simulink model "Commande_2_BackStepping"  (R2015a)
settings: Solver=ode3  StartTime=0.0  StopTime=5  FixedStep=0.0001  RelTol=1e-3
undefined symbols (not defined in the file or in its folder): sfun3d
(part 2 of 2)

== matlab function Commande_2_BackStepping/Point de Foncitonnement/T et ses derivees/Les matrices de lineairisation de d2P   ==
  data: P input; dP input; d2P input; d_d2P_alpha output; d_d2P_dalpha output; d_d2P_d2alpha output
    function [d_d2P_alpha, d_d2P_dalpha, d_d2P_d2alpha ]= fcn(P,dP,d2P)

    l1 = 0.19992; 
    l2 = 0.334; 
    r = 0.126; 
    phi2 = 2*pi/3;
    phi3 = 4*pi/3;

    %% Expression de P dans Ri
    % l'expression P1 dP1 et d2P1 ne se changent pas
    A2=[cos(phi2) sin(phi2) 0
        -sin(phi2) cos(phi2) 0
        0            0      1 ]; 
    A3=[cos(phi3) sin(phi3) 0
        -sin(phi3) cos(phi3) 0
        0            0      1 ];
     P2=A2*P; dP2=A2*dP; d2P2=A2*d2P; 
     P3=A3*P ; dP3=A3*dP ; d2P3=A3*d2P ; 
% Notation        
    x1=P(1); y1=P(2) ; z1=P(3) ; 
    x2=P2(1); y2=P2(2) ; z2=P2(3) ;
    x3=P3(1); y3=P3(2) ; z3=P3(3) ;

    %% Parametres du Triangle AiCiBi :
    % Triangle 1 :
    AB1=sqrt(z1^2+(x1-r)^2);
    e1=sqrt(l2^2-y1^2); 
    AB2=sqrt(z2^2+(x2-r)^2);
    e2=sqrt(l2^2-y2^2);
    AB3=sqrt(z3^2+(x3-r)^2);
    e3=sqrt(l2^2-y3^2);

% calcul de delta1
    delta1=acos((AB1^2 + l1^2 - e1^2)/(2*l1*AB1));
% calcul de delta2
    delta2=acos((AB2^2 + l1^2 - e2^2)/(2*l1*AB2));
% calcul de alpha3
    delta3=acos((AB3^2 + l1^2 - e3^2)/(2*l1*AB3));

%% =================== Calcule de dalpha_i ====================================

% ---------------------------- Calcul de dAlpha1 ----------------------
% Calcule de dDelta1 :
BH1 = AB1-l1*cos(delta1);
D1=l1*AB1*sin(delta1) ;
dDelta1X = -BH1*(x1-r)/AB1/D1 ; 
dDelta1Y = -y1/D1 ; 
dDelta1Z = -BH1*z1/AB1/D1 ; 
Gdelta1=  [ dDelta1X , dDelta1Y , dDelta1Z] ;
% Calcule de dBeta1 :
dBeta1Z=-(x1-r)/AB1^2 ; dBeta1X=z1/AB1^2 ;
Gbeta1=[ dBeta1X ,  0 , dBeta1Z] ;
% Calcule de dAlpha1 :
Galpha1=Gbeta1-Gdelta1 ;

% ---------------------------- Calcul de dAlpha2 ----------------------
% Calcule de dDelta2 :
BH2 = AB2-l1*cos(delta2);
D2=l1*AB2*sin(delta2) ;
dDelta2X = -BH2*(x2-r)/AB2/D2 ; 
dDelta2Y = -y2/D2 ; 
dDelta2Z = -BH2*z2/AB2/D2 ; 
Gdelta2=  [ dDelta2X , dDelta2Y , dDelta2Z] ;
% Calcule de dBeta2 :
dBeta2Z=-(x2-r)/AB2^2 ; dBeta2X=z2/AB2^2 ;
Gbeta2=[ dBeta2X ,  0 , dBeta2Z] ;
% Calcule de dAlpha2 :
Galpha2=Gbeta2-Gdelta2 ;

% ---------------------------- Calcul de dAlpha3 ----------------------
% Calcule de dDelta2 :
BH3 = AB3-l1*cos(delta3);
D3=l1*AB3*sin(delta3) ;
dDelta3X = -BH3*(x3-r)/AB3/D3 ; 
dDelta3Y = -y3/D3 ; 
dDelta3Z = -BH3*z3/AB3/D3 ; 
Gdelta3=  [ dDelta3X , dDelta3Y , dDelta3Z] ;
% Calcule de dBeta3:
dBeta3Z=-(x3-r)/AB3^2 ; dBeta2X=z3/AB3^2 ;
Gbeta3=[ dBeta2X ,  0 , dBeta3Z] ;
% Calcule de dAlpha3 :
Galpha3=Gbeta3-Gdelta3 ;

%% ===================== Calcule de d2alpha_i =================================
 
% ---------------------------- Calcul de d2Alpha1 ----------------------
% Calcule de d2Gama1 :
CH1=l1*sin(delta1);
AH1=l1*cos(delta1) ;
d2Delta1XX = -BH1*(x1-r)^2/(AB1^3*D1)*( AH1*e1^2/(BH1*CH1^2) + (AB1/(x1-r))^2 - 2 ) ;
d2Delta1YY = - (1+y1^2*AH1*AB1/D1^2 )  /D1;
d2Delta1ZZ  = -BH1*z1^2/(AB1^3*D1)*( AH1*e1^2/(BH1*CH1^2) + (AB1/z1)^2 -2 ) ;
d2Delta1XY = y1*(x1-r)*(CH1^2-AH1*BH1)/D1^3 ;
d2Delta1XZ = -BH1*(x1-r)*z1/(AB1^3*D1)*( AH1*e1^2/(BH1*CH1^2) - 2 ) ;
d2Delta1YZ = y1*z1*(CH1^2-AH1*BH1)/D1^3 ; 
Hdelta1=[ d2Delta1XX,d2Delta1XY,d2Delta1XZ ; d2Delta1XY, d2Delta1YY,d2Delta1YZ ;d2Delta1XZ , d2Delta1YZ,d2Delta1ZZ] ;
%Calcule de dBeta 1:
d2Beta1XX=-2*(x1-r)*z1/AB1^4 ; d2Beta1ZZ=-d2Beta1XX ; d2Beta1XZ = ((x1-r)^2-z1^2)/AB1^4 ;
Hbeta1= [d2Beta1XX , 0, d2Beta1XZ ; 0, 0, 0 ; d2Beta1XZ , 0 , d2Beta1ZZ ] ;
%Calcule de dAlpha1 :
Halpha1= Hbeta1 - Hdelta1; 

% ---------------------------- Calcul de d2Alpha2 ----------------------
% Calcule de d2Gama1 :
CH2=l1*sin(delta2);
AH2=l1*cos(delta2) ;
d2Delta2XX = -BH2*(x2-r)^2/(AB2^3*D2)*( AH2*e2^2/(BH2*CH2^2) + (AB2/(x2-r))^2 - 2 ) ;
d2Delta2YY = - (1+y2^2*AH2*AB2/D2^2 )  /D2;
d2Delta2ZZ  = -BH2*z2^2/(AB2^3*D2)*( AH2*e2^2/(BH2*CH2^2) + (AB2/z2)^2 -2 ) ;
d2Delta2XY = y2*(x2-r)*(CH2^2-AH2*BH2)/D2^3 ;
d2Delta2XZ = -BH2*(x2-r)*z2/(AB2^3*D2)*( AH2*e2^2/(BH2*CH2^2) - 2 ) ;
d2Delta2YZ = y2*z2*(CH2^2-AH2*BH2)/D2^3 ; 
Hdelta2=[ d2Delta2XX,d2Delta2XY,d2Delta2XZ ; d2Delta2XY, d2Delta2YY,d2Delta2YZ ;d2Delta2XZ , d2Delta2YZ,d2Delta2ZZ] ;
%Calcule de dBeta2:
d2Beta2XX=-2*(x2-r)*z2/AB2^4 ; d2Beta2ZZ=-d2Beta2XX ; d2Beta2XZ = ((x2-r)^2-z2^2)/AB2^4 ;
Hbeta2= [d2Beta2XX , 0, d2Beta2XZ ; 0, 0, 0 ; d2Beta2XZ , 0 , d2Beta2ZZ ] ;
%Calcule de dAlpha2 :
Halpha2= Hbeta2 - Hdelta2; 

% ---------------------------- Calcul de d2Alpha3 ----------------------
% Calcule de d2Gama3 :
CH3=l1*sin(delta3);
AH3=l1*cos(delta3) ;
d2Delta3XX = -BH3*(x3-r)^2/(AB3^3*D3)*( AH3*e3^2/(BH3*CH3^2) + (AB3/(x3-r))^2 - 2 ) ;
d2Delta3YY = - (1+y3^2*AH3*AB3/D3^2 )  /D3;
d2Delta3ZZ  = -BH3*z3^2/(AB3^3*D3)*( AH3*e3^2/(BH3*CH3^2) + (AB3/z3)^2 -2 ) ;
d2Delta3XY = y3*(x3-r)*(CH3^2-AH3*BH3)/D3^3 ;
d2Delta3XZ = -BH3*(x3-r)*z3/(AB3^3*D3)*( AH3*e3^2/(BH3*CH3^2) - 2 ) ;
d2Delta3YZ = y3*z3*(CH3^2-AH3*BH3)/D3^3 ; 
Hdelta3=[ d2Delta3XX,d2Delta3XY,d2Delta3XZ ; d2Delta3XY, d2Delta3YY,d2Delta3YZ ;d2Delta3XZ , d2Delta3YZ,d2Delta3ZZ] ;
%Calcule de dBeta3:
d2Beta3XX=-2*(x3-r)*z3/AB3^4 ; d2Beta3ZZ=-d2Beta3XX ; d2Beta3XZ = ((x3-r)^2-z3^2)/AB3^4 ;
Hbeta3= [d2Beta3XX , 0, d2Beta3XZ ; 0, 0, 0 ; d2Beta3XZ , 0 , d2Beta3ZZ ] ;
%Calcule de dAlpha3 :
Halpha3= Hbeta3 - Hdelta3; 

%% ==================== Caclcule de d3Alpahi ==================

%% ------------------------------ 1)  Calcule de d3Alpha1 -----------------------------
% Calcule de d3Delta1 :
% Parametres (1er derivees):
DH1=CH1^2-AH1*BH1 ;
dAB1X=(x1-r)/AB1 ; dAB1Z = z1/AB1 ; 
dD1X=(x1-r)*DH1/D1 ; dD1Z= z1*DH1/D1; dD1Y=-y1*AH1/CH1 ;
dAH1X=(x1-r)*BH1/AB1^2 ; dAH1Z = z1*BH1/AB1^2  ; 
dBH1X=(x1-r)*AH1/AB1^2 ; dBH1Z = z1*AH1/AB1^2  ; 
% Parametres (2eme derivees partielles):
% d2D1
d2D1XX=(DH1-(x1-r)^2-(dD1X)^2)/D1 ;
d2D1ZZ=(DH1-z1^2-(dD1Z)^2)/D1 ;
d2D1YY= -AH1/CH1-y1^2/D1*(1+(AH1/CH1)^2);
d2D1XZ = -(z1*(x1-r) + dD1X*dD1Z)/D1 ;
% d2AB1
d2AB1XX = 1/AB1 - (x1-r)*dAB1X/AB1^2 ;
d2AB1ZZ= 1/AB1 - z1*dAB1Z/AB1^2 ;
d2AB1XZ=-z1*(x1-r)/AB1^3;
%d2BH1
d2BH1ZZ=dBH1Z*(dAH1Z/AH1 +1/z1 - 2*dAB1Z/AB1) ;
d2BH1XX=dBH1X*(dAH1X/AH1 +1/(x1-r) - 2*dAB1X/AB1) ;
d2BH1XZ=z1*(x1-r)*(BH1-2*AH1)/AB1^4 ;

%------------------- les derivees partielles  d3Delta1_
d3Delta1ZZZ = d2Delta1ZZ*(dBH1Z/BH1+1/z1-dAB1Z/AB1-dD1Z/D1) + dDelta1Z*(-(dBH1Z/BH1)^2-1/z1^2+(dAB1Z/AB1)^2+(dD1Z/D1)^2 + d2BH1ZZ/BH1 - d2AB1ZZ/AB1 -d2D1ZZ/D1);
d3Delta1XXX = d2Delta1XX*(dBH1X/BH1+1/(x1-r)-dAB1X/AB1-dD1X/D1) + dDelta1X*(-(dBH1X/BH1)^2-1/(x1-r)^2+(dAB1X/AB1)^2+(dD1X/D1)^2 + d2BH1XX/BH1 - d2AB1XX/AB1 -d2D1XX/D1);
d3Delta1YYY= dD1Y/D1^2 + D1^2\(dD1Y + y1*d2D1YY-2*(dD1Y)^2*y1/D1);
d3Delta1XZZ= d2Delta1XZ*(dBH1Z/BH1+1/z1-dAB1Z/AB1-dD1Z/D1)+dDelta1Z*(-dBH1X*dBH1Z/BH1^2 + dAB1Z*dAB1X/AB1^2 + dD1Z*dD1X/D1^2 + d2BH1XZ/BH1 - d2AB1XZ/AB1 -d2D1XZ/D1) ;
d3Delta1XXZ= d2Delta1XZ*(dBH1X/BH1+1/(x1-r)-dAB1X/AB1-dD1X/D1)+dDelta1X*(-dBH1X*dBH1Z/BH1^2 + dAB1Z*dAB1X/AB1^2 + dD1Z*dD1X/D1^2 + d2BH1XZ/BH1 - d2AB1XZ/AB1 -d2D1XZ/D1) ;
d3Delta1XYY=(x1-r)/D1^3*(DH1-y1^2-3*y1*DH1*dD1Y/D1);
d3Delta1XXY=y1/D1^3*(DH1-(x1-r)^2*(1+3*(DH1/D1)^2));
d3Delta1YYZ=z1/D1^3*(DH1-y1^2-3*y1*DH1*dD1Y/D1);
d3Delta1YZZ=y1/D1^3*(DH1-z1^2*(1+3*(DH1/D1)^2));
d3Delta1XYZ=-(x1-r)*y1*z1/D1^3*(1+3*(DH1/D1)^2);
dHdelta1X=[ d3Delta1XXX,d3Delta1XXY,d3Delta1XXZ ; d3Delta1XXY, d3Delta1XYY,d3Delta1XYZ ;d3Delta1XXZ , d3Delta1XYZ,d3Delta1XZZ] ;
dHdelta1Y=[ d3Delta1XXY,d3Delta1XYY,d3Delta1XYZ ; d3Delta1XYY, d3Delta1YYY,d3Delta1YYZ ;d3Delta1XYZ , d3Delta1YYZ,d3Delta1YZZ] ;
dHdelta1Z=[ d3Delta1XXZ,d3Delta1XYZ,d3Delta1XZZ ; d3Delta1XYZ, d3Delta1YYZ,d3Delta1YZZ ;d3Delta1XZZ , d3Delta1YZZ,d3Delta1ZZZ] ;
%d3Delta1= 3*dP'*Hdelta1*d2P + Gdelta1*d3P + dP'*[dHdelta1X*dP,dHdelta1Y*dP , dHdelta1Z*dP]*dP ;
%---------------  les derivees partielles  d3Beta1_
d3Beta1XXX=-2*z1/AB1^4*(1-4*((x1-r)/AB1)^2) ; 
d3Beta1ZZZ=2*(x1-r)/AB1^4*(1-4*(z1/AB1)^2) ; 
d3Beta1XZZ=-d3Beta1XXX;d3Beta1XXZ=-d3Beta1ZZZ ;
dHbeta1X=[d3Beta1XXX , 0 ,d3Beta1XXZ ; 0,0,0;d3Beta1XXZ , 0 , d3Beta1XZZ];
dHbeta1Z=[d3Beta1XXZ , 0 ,d3Beta1XZZ ; 0,0,0;d3Beta1XZZ , 0 , d3Beta1ZZZ];
dHbeta1Y= zeros(3) ;
%d3Beta1=3*dP'*Hbeta1*d2P + Gbeta1*d3P + dP'*[dHbeta1X*dP,dHbeta1Y*dP, dHbeta1Z*dP]*dP ;
% En fin :
dHalpha1X=dHbeta1X-dHdelta1X ;
dHalpha1Y=dHbeta1Y-dHdelta1Y ;
dHalpha1Z=dHbeta1Z-dHdelta1Z ;
%d3Alpha1=3*dP'*Halpha1*d2P + Galpha1*d3P + dP'*[dHalpha1X*dP,dHalpha1Y*dP, dHalpha1Z*dP]*dP ;
%% -------------------------------2) Calcule de d3Alpha2 -----------------------------
% Calcule de d3Delta2 :
% Parametres (1er derivees):
DH2=CH2^2-AH2*BH2 ;
dAB2X=(x2-r)/AB2 ; dAB2Z = z2/AB2 ; 
dD2X=(x2-r)*DH2/D2 ; dD2Z= z2*DH2/D2; dD2Y=-y2*AH2/CH2 ;
dAH2X=(x2-r)*BH2/AB2^2 ; dAH2Z = z2*BH2/AB2^2  ; 
dBH2X=(x2-r)*AH2/AB2^2 ; dBH2Z = z2*AH2/AB2^2  ; 
% Parametres (2eme derivees partielles):
% d2D2
d2D2XX=(DH2-(x2-r)^2-(dD2X)^2)/D2 ;
d2D2ZZ=(DH2-z2^2-(dD2Z)^2)/D2 ;
d2D2YY= -AH2/CH2-y2^2/D2*(1+(AH2/CH2)^2);
d2D2XZ = -(z2*(x2-r) + dD2X*dD2Z)/D2 ;
% d2AB2
d2AB2XX = 1/AB2 - (x2-r)*dAB2X/AB2^2 ;
d2AB2ZZ= 1/AB2 - z2*dAB2Z/AB2^2 ;
d2AB2XZ=-z2*(x2-r)/AB2^3;
%d2BH2
d2BH2ZZ=dBH2Z*(dAH2Z/AH2 +1/z2 - 2*dAB2Z/AB2) ;
d2BH2XX=dBH2X*(dAH2X/AH2 +1/(x2-r) - 2*dAB2X/AB2) ;
d2BH2XZ=z2*(x2-r)*(BH2-2*AH2)/AB2^4 ;

%------------- les derivees partielles  d3Delta1_
d3Delta2ZZZ = d2Delta2ZZ*(dBH2Z/BH2+1/z2-dAB2Z/AB2-dD2Z/D2) + dDelta2Z*(-(dBH2Z/BH2)^2-1/z2^2+(dAB2Z/AB2)^2+(dD2Z/D2)^2 + d2BH2ZZ/BH2 - d2AB2ZZ/AB2 -d2D2ZZ/D2);
d3Delta2XXX = d2Delta2XX*(dBH2X/BH2+1/(x2-r)-dAB2X/AB2-dD2X/D2) + dDelta2X*(-(dBH2X/BH2)^2-1/(x2-r)^2+(dAB2X/AB2)^2+(dD2X/D2)^2 + d2BH2XX/BH2 - d2AB2XX/AB2 -d2D2XX/D2);
d3Delta2YYY= dD2Y/D2^2 + D2^2\(dD2Y + y2*d2D2YY-2*(dD2Y)^2*y2/D2);
d3Delta2XZZ= d2Delta2XZ*(dBH2Z/BH2+1/z2-dAB2Z/AB2-dD2Z/D2)+dDelta2Z*(-dBH2X*dBH2Z/BH2^2 + dAB2Z*dAB2X/AB2^2 + dD2Z*dD2X/D2^2 + d2BH2XZ/BH2 - d2AB2XZ/AB2 -d2D2XZ/D2) ;
d3Delta2XXZ= d2Delta2XZ*(dBH2X/BH2+1/(x2-r)-dAB2X/AB2-dD2X/D2)+dDelta2X*(-dBH2X*dBH2Z/BH2^2 + dAB2Z*dAB2X/AB2^2 + dD2Z*dD2X/D2^2 + d2BH2XZ/BH2 - d2AB2XZ/AB2 -d2D2XZ/D2) ;
d3Delta2XYY=(x2-r)/D2^3*(DH2-y2^2-3*y2*DH2*dD2Y/D2);
d3Delta2XXY=y2/D2^3*(DH2-(x2-r)^2*(1+3*(DH2/D2)^2));
d3Delta2YYZ=z2/D2^3*(DH2-y2^2-3*y2*DH2*dD2Y/D2);
d3Delta2YZZ=y2/D2^3*(DH2-z2^2*(1+3*(DH2/D2)^2));
d3Delta2XYZ=-(x2-r)*y2*z2/D2^3*(1+3*(DH2/D2)^2);
dHdelta2X=[ d3Delta2XXX,d3Delta2XXY,d3Delta2XXZ ; d3Delta2XXY, d3Delta2XYY,d3Delta2XYZ ;d3Delta2XXZ , d3Delta2XYZ,d3Delta2XZZ] ;
dHdelta2Y=[ d3Delta2XXY,d3Delta2XYY,d3Delta2XYZ ; d3Delta2XYY, d3Delta2YYY,d3Delta2YYZ ;d3Delta2XYZ , d3Delta2YYZ,d3Delta2YZZ] ;
dHdelta2Z=[ d3Delta2XXZ,d3Delta2XYZ,d3Delta2XZZ ; d3Delta2XYZ, d3Delta2YYZ,d3Delta2YZZ ;d3Delta2XZZ , d3Delta2YZZ,d3Delta2ZZZ] ;
%%  les derivees partielles  d3Beta2_
d3Beta2XXX=-2*z2/AB2^4*(1-4*((x2-r)/AB2)^2) ; 
d3Beta2ZZZ=2*(x2-r)/AB2^4*(1-4*(z2/AB2)^2) ; 
d3Beta2XZZ=-d3Beta2XXX;d3Beta1XXZ=-d3Beta2ZZZ ;
dHbeta2X=[d3Beta2XXX , 0 ,d3Beta1XXZ ; 0,0,0;d3Beta1XXZ , 0 , d3Beta2XZZ];
dHbeta2Z=[d3Beta1XXZ , 0 ,d3Beta2XZZ ; 0,0,0;d3Beta2XZZ , 0 , d3Beta2ZZZ];
dHbeta2Y= zeros(3) ;
% En fin :
dHalpha2X=dHbeta2X-dHdelta2X ;
dHalpha2Y=dHbeta2Y-dHdelta2Y ;
dHalpha2Z=dHbeta2Z-dHdelta2Z ;

%% -------------------------------3) Calcule de d3Alpha3 -----------------------------
% Calcule de d3Delta3 :
% Parametres (1er derivees):
DH3=CH3^2-AH3*BH3 ;
dAB3X=(x3-r)/AB3 ; dAB3Z = z3/AB3 ; 
dD3X=(x3-r)*DH3/D3 ; dD3Z= z3*DH3/D3; dD3Y=-y3*AH3/CH3 ;
dAH3X=(x3-r)*BH3/AB3^2 ; dAH3Z = z3*BH3/AB3^2  ; 
dBH3X=(x3-r)*AH3/AB3^2 ; dBH3Z = z3*AH3/AB3^2  ; 

% Parametres (2eme derivees partielles):
% d2D3
d2D3XX=(DH3-(x3-r)^2-(dD3X)^2)/D3 ;
d2D3ZZ=(DH3-z3^2-(dD3Z)^2)/D3 ;
d2D3YY= -AH3/CH3-y3^2/D3*(1+(AH3/CH3)^2);
d2D3XZ = -(z3*(x3-r) + dD3X*dD3Z)/D3 ;
% d2AB3
d2AB3XX = 1/AB3 - (x3-r)*dAB3X/AB3^2 ;
d2AB3ZZ= 1/AB3 - z3*dAB3Z/AB3^2 ;
d2AB3XZ=-z3*(x3-r)/AB3^3;
%d2BH3
d2BH3ZZ=dBH3Z*(dAH3Z/AH3 +1/z3 - 2*dAB3Z/AB3) ;
d2BH3XX=dBH3X*(dAH3X/AH3 +1/(x3-r) - 2*dAB3X/AB3) ;
d2BH3XZ=z3*(x3-r)*(BH3-2*AH3)/AB3^4 ;


%%  les derivees partielles  d3Delta3_
d3Delta3ZZZ = d2Delta3ZZ*(dBH3Z/BH3+1/z3-dAB3Z/AB3-dD3Z/D3) + dDelta3Z*(-(dBH3Z/BH3)^2-1/z3^2+(dAB3Z/AB3)^2+(dD3Z/D3)^2 + d2BH3ZZ/BH3 - d2AB3ZZ/AB3 -d2D3ZZ/D3);
d3Delta3XXX = d2Delta3XX*(dBH3X/BH3+1/(x3-r)-dAB3X/AB3-dD3X/D3) + dDelta3X*(-(dBH3X/BH3)^2-1/(x3-r)^2+(dAB3X/AB3)^2+(dD3X/D3)^2 + d2BH3XX/BH3 - d2AB3XX/AB3 -d2D3XX/D3);
d3Delta3YYY= dD3Y/D3^2 + D3^2\(dD3Y + y3*d2D3YY-2*(dD3Y)^2*y3/D3);
d3Delta3XZZ= d2Delta3XZ*(dBH3Z/BH3+1/z3-dAB3Z/AB3-dD3Z/D3)+dDelta3Z*(-dBH3X*dBH3Z/BH3^2 + dAB3Z*dAB3X/AB3^2 + dD3Z*dD3X/D3^2 + d2BH3XZ/BH3 - d2AB3XZ/AB3 -d2D3XZ/D3) ;
d3Delta3XXZ= d2Delta3XZ*(dBH3X/BH3+1/(x3-r)-dAB3X/AB3-dD3X/D3)+dDelta3X*(-dBH3X*dBH3Z/BH3^2 + dAB3Z*dAB3X/AB3^2 + dD3Z*dD3X/D3^2 + d2BH3XZ/BH3 - d2AB3XZ/AB3 -d2D3XZ/D3) ;
d3Delta3XYY=(x3-r)/D3^3*(DH3-y3^2-3*y3*DH3*dD3Y/D3);
d3Delta3XXY=y3/D3^3*(DH3-(x3-r)^2*(1+3*(DH3/D3)^2));
d3Delta3YYZ=z3/D3^3*(DH3-y3^2-3*y3*DH3*dD3Y/D3);
d3Delta3YZZ=y3/D3^3*(DH3-z3^2*(1+3*(DH3/D3)^2));
d3Delta3XYZ=-(x3-r)*y3*z3/D3^3*(1+3*(DH3/D3)^2);
dHdelta3X=[ d3Delta3XXX,d3Delta3XXY,d3Delta3XXZ ; d3Delta3XXY, d3Delta3XYY,d3Delta3XYZ ;d3Delta3XXZ , d3Delta3XYZ,d3Delta3XZZ] ;
dHdelta3Y=[ d3Delta3XXY,d3Delta3XYY,d3Delta3XYZ ; d3Delta3XYY, d3Delta3YYY,d3Delta3YYZ ;d3Delta3XYZ , d3Delta3YYZ,d3Delta3YZZ] ;
dHdelta3Z=[ d3Delta3XXZ,d3Delta3XYZ,d3Delta3XZZ ; d3Delta3XYZ, d3Delta3YYZ,d3Delta3YZZ ;d3Delta3XZZ , d3Delta3YZZ,d3Delta3ZZZ] ;
%--------------  les derivees partielles  d3Beta3_
d3Beta3XXX=-2*z3/AB3^4*(1-4*((x3-r)/AB3)^2) ; 
d3Beta3ZZZ=2*(x3-r)/AB3^4*(1-4*(z3/AB3)^2) ; 
d3Beta3XZZ=-d3Beta3XXX;d3Beta1XXZ=-d3Beta3ZZZ ;
dHbeta3X=[d3Beta3XXX , 0 ,d3Beta1XXZ ; 0,0,0;d3Beta1XXZ , 0 , d3Beta3XZZ];
dHbeta3Z=[d3Beta1XXZ , 0 ,d3Beta3XZZ ; 0,0,0;d3Beta3XZZ , 0 , d3Beta3ZZZ];
dHbeta3Y= zeros(3) ;
% En fin :
dHalpha3X=dHbeta3X-dHdelta3X ;
dHalpha3Y=dHbeta3Y-dHdelta3Y ;
dHalpha3Z=dHbeta3Z-dHdelta3Z ;

%% |||||||||||||||||||||||=====================================|||||||||||||||||||||
%%                             Calcule de : d_d2P_alpha , d_d2P_dalpha ,et d_d2P_d2alpha
%% |||||||||||||||||||||||||||===========================|||||||||||||||||||||||||||

    % Notaion :
    % d_d2P_alpha : C'est la derivee partielle de d2P par rapport au alpha
    % d_d2P_dalpha : C'est la derivee partielle de d2P par rapport au dalpha
    % d_d2P_d2alpha : C'est la derivee partielle de d2P par rapport au d2alpha
    % dP_j_i : C'est la derivee partielle de P_j par rapport au alpha _i
    % dGalpha_j_i : C'est la derivee partielle du Gradient de alpha_j par rapport au alpha _i
    % dHalpha_j_i : C'est la derivee partielle de la matricr hessienne_j par rapport au alpha _i
    % d_dP_alpha : C'est la derivee partielle de la vitesse dP par rapport au alpha
% Parametres :
    E1=[1 0 0] ; E2=[0 1 0] ; E3=[0 0 1] ;

% A) Calcule de J
    J = [Galpha1 ; Galpha2*A2 ; Galpha3*A3] ;

% B) Calcule de dP_j_i
    dP1_1=J\E1' ; dP1_2=J\E2' ; dP1_3=J\E3' ;
    dP2_1=A2*dP1_1 ; dP2_2=A2*dP1_2; dP2_3= A2*dP1_3;
    dP3_1=A3*dP1_1 ; dP3_2=A3*dP1_2; dP3_3= A3*dP1_3;

% B) Calcule de dGalpha_j_i
     dGalpha1_1=dP1_1'*Halpha1 ; dGalpha1_2=dP1_2'*Halpha1 ; dGalpha1_3 = dP1_3'*Halpha1 ;
     dGalpha2_1=dP2_1'*Halpha2 ; dGalpha2_2=dP2_2'*Halpha2 ; dGalpha2_3 = dP2_3'*Halpha2 ;
     dGalpha3_1=dP3_1'*Halpha3 ; dGalpha3_2=dP3_2'*Halpha3 ; dGalpha3_3 = dP3_3'*Halpha3 ;
 
 % C) Calcule de dHalpha_j_i 
     % 1) les derivee de Halpha1
     dHalpha1_1=dHalpha1X*(E1*dP1_1) + dHalpha1Y*(E2*dP1_1)+dHalpha1Z*(E3*dP1_1) ;
     dHalpha1_2=dHalpha1X*(E1*dP1_2) + dHalpha1Y*(E2*dP1_2)+dHalpha1Z*(E3*dP1_2) ;
     dHalpha1_3=dHalpha1X*(E1*dP1_3) + dHalpha1Y*(E2*dP1_3)+dHalpha1Z*(E3*dP1_3) ;
     % 2) les derivee de Halpha2
     dHalpha2_1=dHalpha2X*(E1*dP2_1 )+ dHalpha2Y*(E2*dP2_1)+dHalpha2Z*(E3*dP2_1) ;
     dHalpha2_2=dHalpha2X*(E1*dP2_2 )+ dHalpha2Y*(E2*dP2_2)+dHalpha2Z*(E3*dP2_2) ;
     dHalpha2_3=dHalpha2X*(E1*dP2_3 )+ dHalpha2Y*(E2*dP2_3)+dHalpha2Z*(E3*dP2_3) ;
     % 3) les derivee de Halpha3
     dHalpha3_1=dHalpha3X*(E1*dP3_1) + dHalpha3Y*(E2*dP3_1)+dHalpha3Z*(E3*dP3_1) ;
     dHalpha3_2=dHalpha3X*(E1*dP3_2) + dHalpha3Y*(E2*dP3_2)+dHalpha3Z*(E3*dP3_2) ;
     dHalpha3_3=dHalpha3X*(E1*dP3_3) + dHalpha3Y*(E2*dP3_3)+dHalpha3Z*(E3*dP3_3) ;
     
%D) Calcule de ddPalpha
    d_dP_alpha=-J\[dP'*Halpha1 ; dP2'*Halpha2*A2 ; dP3'*Halpha3*A3]/J ;
    
% E) Calcule de coefficients ai_j :
    a11 = 2*dP'*Halpha1*d_dP_alpha(:,1) + dP'*dHalpha1_1*dP + dGalpha1_1*d2P;
    a21 = 2*dP'*Halpha1*d_dP_alpha(:,2) + dP'*dHalpha1_2*dP + dGalpha1_2*d2P;
    a31 = 2*dP'*Halpha1*d_dP_alpha(:,3) + dP'*dHalpha1_3*dP + dGalpha1_3*d2P;
    %
    a12 = 2*dP2'*Halpha2*A2*d_dP_alpha(:,1) + dP2'*dHalpha2_1*dP2 + dGalpha2_1*d2P2;
    a22 = 2*dP2'*Halpha2*A2*d_dP_alpha(:,2) + dP2'*dHalpha2_2*dP2 + dGalpha2_2*d2P2;
    a32 = 2*dP2'*Halpha2*A2*d_dP_alpha(:,3) + dP2'*dHalpha2_3*dP2 + dGalpha2_3*d2P2;
    %
    a13 = 2*dP3'*Halpha3*A3*d_dP_alpha(:,1) + dP3'*dHalpha3_1*dP3 + dGalpha3_1*d2P3;
    a23 = 2*dP3'*Halpha3*A3*d_dP_alpha(:,2) + dP3'*dHalpha3_2*dP3 + dGalpha3_2*d2P3;
    a33 = 2*dP3'*Halpha3*A3*d_dP_alpha(:,3) + dP3'*dHalpha3_3*dP3 + dGalpha3_3*d2P3;
    
% F) Calcule de d_d2P_alpha 
    d_d2P_alpha = -J\[a11 , a21 , a31 ; a12 , a22 , a32 ; a13 , a23 , a33];
    
% G) Calcule de d_d2P_dalpha_i
    d_d2P_dalpha1 = -J\[ dP1_1'*Halpha1*dP ; dP2_1'*Halpha2*dP2 ; dP3_1'*Halpha3*dP3] -J\[ dP'*Halpha1*dP1_1; dP2'*Halpha2*dP2_1 ; dP3'*Halpha3*dP3_1] ;
    d_d2P_dalpha2 = -J\[ dP1_2'*Halpha1*dP ; dP2_2'*Halpha2*dP2 ; dP3_2'*Halpha3*dP3]-J\[ dP'*Halpha1*dP1_2 ; dP2'*Halpha2*dP2_2 ; dP3'*Halpha3*dP3_2] ;
    d_d2P_dalpha3 = -J\[ dP1_3'*Halpha1*dP ; dP2_3'*Halpha2*dP2 ; dP3_3'*Halpha3*dP3]-J\[ dP'*Halpha1*dP1_3 ; dP2'*Halpha2*dP2_3 ; dP3'*Halpha3*dP3_3] ;
    d_d2P_dalpha = [d_d2P_dalpha1 , d_d2P_dalpha2 , d_d2P_dalpha3] ;

% K) Calcule de d_d2P_d2alpha_i :
    d_d2P_d2alpha = eye(3)/J ;
    
% L) verification :
    %d3P1 = d_d2P_alpha* dalpha + d_d2P_dalpha*  d2alpha  + d_d2P_d2alpha*  d3alpha;

== matlab function Commande_2_BackStepping/Point de Foncitonnement/T et ses derivees/dCai par derivees partielles  ==
  data: T output; dT output; Tg input; dTg_Theta input; P input; d2P input; alpha input; dalpha input; d2alpha input; d3alpha input; d_d2P_alpha input; d_d2P_dalpha input; d_d2P_d2alpha input; dT_Theta output; dT_dTheta output; dT_d2Theta output
function [T,dT,dT_Theta,dT_dTheta,dT_d2Theta] = fcn(Tg,dTg_Theta ,P,d2P,alpha,dalpha,d2alpha,d3alpha,d_d2P_alpha, d_d2P_dalpha, d_d2P_d2alpha)

alpha1=alpha(1) ;alpha2=alpha(2) ; alpha3=alpha(3) ;
dalpha1=dalpha(1) ;dalpha2=dalpha(2) ; dalpha3=dalpha(3) ;
d2alpha1=d2alpha(1) ;d2alpha2=d2alpha(2) ; d2alpha3=d2alpha(3) ;

%% les constantes
    l1 = 0.19992; 
    l2 = 0.334; 
    r = 0.126; 
    phi2 = 2*pi/3;
    phi3 = 4*pi/3;
A2=[cos(phi2) sin(phi2) 0
    -sin(phi2) cos(phi2) 0
    0            0      1 ]; 
A3=[cos(phi3) sin(phi3) 0
    -sin(phi3) cos(phi3) 0
    0            0      1 ];
% Constantes mecaniques
    J1=0.0071126;
    M2=2*0.01438  ;
    J2 = 2*0.00027499613;
    M3 = 0.04157 ;
    M4=2*J2/l2^2 ;
    
% Fin

% les vecteurs OAi et OCi :
OC1=[r+l1*cos(alpha1) ; 0 ; -l1*sin(alpha1) ]; 
OC2=[(r+l1*cos(alpha2))*cos(phi2) ; (r+l1*cos(alpha2))*sin(phi2) ; -l1*sin(alpha2) ]; 
OC3=[(r+l1*cos(alpha3))*cos(phi3) ; (r+l1*cos(alpha3))*sin(phi3) ; -l1*sin(alpha3) ]; 
%fin

% Les vecteurs unitaires portes par les bras paralleles : la nouvelle base
u1=(P-OC1)/l2 ; u2=(P-OC2)/l2 ; u3=(P-OC3)/l2 ;
%la matrice du transformation = La nouvelle base:
U = [u1 u2 u3] ;
Uinv = eye(3)/U ;
%Uinv=inv(U);

%%  accelerations des points Ci :
% dOCi : la derivee partielle de OCi par rapport au alphai
% d2OCi : la deuxieme derivee partielle de OCi par rapport au alphai

dOC1_1=[-l1*sin(alpha1) ; 0 ; -l1*cos(alpha1)] ; 
dOC2_2=[-l1*sin(alpha2)*cos(phi2) ; -l1*sin(alpha2)*sin(phi2) ; -l1*cos(alpha2)] ;
dOC3_3=[-l1*sin(alpha3)*cos(phi3) ; -l1*sin(alpha3)*sin(phi3) ; -l1*cos(alpha3)] ;

d2OC1_1=[-l1*cos(alpha1) ; 0 ; l1*sin(alpha1)] ;
d2OC2_2=[-l1*cos(alpha2)*cos(phi2) ; -l1*cos(alpha2)*sin(phi2) ; l1*sin(alpha2)] ;
d2OC3_3=[-l1*cos(alpha3)*cos(phi3) ; -l1*cos(alpha3)*sin(phi3) ; l1*sin(alpha3)] ;

d2OC1 = d2OC1_1*dalpha1^2 + dOC1_1*d2alpha1;
d2OC2 = d2OC2_2*dalpha2^2 + dOC2_2*d2alpha2;
d2OC3 = d2OC3_3*dalpha3^2 + dOC3_3*d2alpha3;
%Fin

%% ================ Le couple Cai en point de fonctionnement Couple1==================
% Parametres:
a1 = M2/4-M4/2 ; a2= M2/4 + M4/2; a3=M3 +3*a2 ; 
% la matrice de cross(AiCi,...)=aci  "ACi est exprimee dans le repere Ri"
ac1=[ 0 , l1*sin(alpha1) , 0 ; -l1*sin(alpha1) ,0 , -l1*cos(alpha1) ; 0 , l1*cos(alpha1),0]   ;
ac2=[ 0 , l1*sin(alpha2) , 0 ; -l1*sin(alpha2) ,0 , -l1*cos(alpha2) ; 0 , l1*cos(alpha2),0]   ;
ac3=[ 0 , l1*sin(alpha3) , 0 ; -l1*sin(alpha3) ,0 , -l1*cos(alpha3) ; 0 , l1*cos(alpha3),0]   ;
% Les matrices de projection
E1 = [1 0 0]; E2 = [0 1 0]; E3 = [0 0 1];
B1= [1 0 0; 0 0 0 ; 0 0 1] ; B2=B1*A2; B3=B1*A3 ;
%% 1)  Le couple Ca1 : 
G11=a3*(E2*ac1*B1*u1)*(E1/U) + a1*E2*ac1*B1 ;
G12=a1*(E2*ac1*B1*u1)*(E1/U)  ;
G13=a1*(E2*ac1*B1*u1)*(E1/U) + a2*E2*ac1*B1 ;
Ca1=(J1+G13*dOC1_1)*d2alpha1+ G11*d2P +(G12*dOC2_2)*d2alpha2 + (G12*dOC3_3)*d2alpha3 +G13*d2OC1_1*dalpha1^2+ (G12*d2OC2_2)*dalpha2^2 + (G12*d2OC3_3)*dalpha3^2;
% Ca1 = J1*d2alpha1 + G11*d2P + G12* (d2OC2 +d2OC3) + G13*d2OC1 ;

%% 2)  Le couple Ca2 : 
G21=a3*(E2*ac2*B2*u2)*(E2/U) + a1*E2*ac2*B2 ;
G22=a1*(E2*ac2*B2*u2)*(E2/U)  ;
G23=a1*(E2*ac2*B2*u2)*(E2/U) + a2*E2*ac2*B2 ;
Ca2=(J1+G23*dOC2_2)*d2alpha2+ G21*d2P +(G22*dOC1_1)*d2alpha1 + (G22*dOC3_3)*d2alpha3 +G23*d2OC2_2*dalpha2^2+ (G22*d2OC1_1)*dalpha1^2 + (G22*d2OC3_3)*dalpha3^2;
%Ca2 = J1*d2alpha2 + G21*d2P + G22* (d2OC1 +d2OC3) + G23*d2OC2 ;

%% 3)  Le couple Ca3 : 
G31=a3*(E2*ac3*B3*u3)*(E3/U) + a1*E2*ac3*B3 ;
G32=a1*(E2*ac3*B3*u3)*(E3/U)  ;
G33=a1*(E2*ac3*B3*u3)*(E3/U) + a2*E2*ac3*B3 ;
Ca3=(J1+G33*dOC3_3)*d2alpha3+ G31*d2P +(G32*dOC2_2)*d2alpha2 + (G32*dOC1_1)*d2alpha1 + G33*d2OC3_3*dalpha3^2+ (G32*d2OC2_2)*dalpha2^2 + (G32*d2OC1_1)*dalpha1^2;
% Ca3 = J1*d2alpha3 + G31*d2P + G32* (d2OC2 +d2OC1) + G33*d2OC3 ;
% Fin
 
Ca = [Ca1 ; Ca2 ; Ca3 ];
Ta=Ca /12 ;

%% ||||||||||||||||||||||||||||||||||||||||||||||||||||||||||||||||
%%         ==== Linearisation de Cai en point de fonctionnement =====
%% ||||||||||||||||||||||||||||||||||||||||||||||||||||||||||||||||

% Notation
% d_d2OCj_alpha_i : C'est la derivee partielle de d2OCj par rapport au alpha i
% dG11_i : C'est la derivee partielle de G11 par rapport au alpha i
% dU_i : la derivee partielle de la matrice U par rapport au alpha i
% duj_i : la derivee partielle du vecteur uj par rapport au alphai
% dACi_i : la derivee partielle de la matrice ACi par rapport au alpha i


% A1)  les derivees partielles de la matrice U  par rapport au Alpha_i
Jinv = d_d2P_d2alpha;
du1_1=(Jinv*E1'-dOC1_1)/l2 ; 
du1_2=(Jinv*E2')/l2 ; 
du1_3=(Jinv*E3')/l2 ;
du2_1=(Jinv*E1')/l2 ;
du2_2=(Jinv*E2'-dOC2_2)/l2 ; 
du2_3=du1_3 ;
du3_1=du2_1; 
du3_2=du1_2; 
du3_3=(Jinv*E3'-dOC3_3)/l2 ;
% En fin
dU_1=[du1_1 , du2_1 , du3_1];  dUinv_1=-Uinv*dU_1*Uinv ;
dU_2=[du1_2 , du2_2 , du3_2]; dUinv_2=-Uinv*dU_2*Uinv ;
dU_3=[du1_3 , du2_3 , du3_3]; dUinv_3=-Uinv*dU_3*Uinv ;
%dU=dU_1*dalpha1+dU_2*dalpha2+dU_3*dalpha3 ;
%dUinv=dUinv_1*dalpha1+dUinv_2*dalpha2+dUinv_3*dalpha3 ;

% A2) Calcule de d_d2OCj_alpha_i :
d_d2OC1_alpha1 = d2OC1_1*d2alpha1- dalpha1^2*dOC1_1 ;
d_d2OC2_alpha2 = d2OC2_2*d2alpha2- dalpha2^2*dOC2_2 ;
d_d2OC3_alpha3 = d2OC3_3*d2alpha3- dalpha3^2*dOC3_3 ;

% A3) Caclcule de d_d2P_alpha i
d_d2P_alpha1 = d_d2P_alpha(:, 1) ;
d_d2P_alpha2 = d_d2P_alpha(:, 2) ;
d_d2P_alpha3 = d_d2P_alpha(:, 3) ;

% A4) Caclcule de d_d2P_dalpha i
d_d2P_dalpha1 = d_d2P_dalpha(:, 1) ;
d_d2P_dalpha2 = d_d2P_dalpha(:, 2) ;
d_d2P_dalpha3 = d_d2P_dalpha(:, 3) ;

% A5) Caclcule de d_d2P_dalpha i
d_d2P_d2alpha1 = d_d2P_d2alpha(:, 1) ;
d_d2P_d2alpha2 = d_d2P_d2alpha(:, 2) ;
d_d2P_d2alpha3 = d_d2P_d2alpha(:, 3) ;
%d3P1 = d_d2P_alpha* dalpha0 + d_d2P_dalpha*  d2alpha0  + d_d2P_d2alpha*  d3alpha;

%% ----------------------------- Linreairisation de Ca1 --------------------------------------

% A) la derivee de aci par rapport au ac1 :
dac1_1=[         0             l1*cos(alpha1)           0 
        -l1*cos(alpha1)            0             l1*sin(alpha1) 
                 0              -l1*sin(alpha1)          0                 ]   ;   

% B) Calcule de dG11_i
dG11_1 = a3*(E2*dac1_1*B1*u1 +E2*ac1*B1*du1_1)*(E1*Uinv) + a3*(E2*ac1*B1*u1)*(E1*dUinv_1) + a1*E2*dac1_1*B1 ;
dG11_2 = a3*(E2*ac1*B1*du1_2)*(E1*Uinv) + a3*(E2*ac1*B1*u1)*(E1*dUinv_2) ;
dG11_3 = a3*(E2*ac1*B1*du1_3)*(E1*Uinv) + a3*(E2*ac1*B1*u1)*(E1*dUinv_3) ;
%dG11= dG11_1*dalpha1 + dG11_2*dalpha2 + dG11_3*dalpha3 ;

% C) Calcule de dG12_i
dG12_1 = a1*(E2*dac1_1*B1*u1 +E2*ac1*B1*du1_1)*(E1*Uinv) + a1*(E2*ac1*B1*u1)*(E1*dUinv_1) ;
dG12_2 = a1*(E2*ac1*B1*du1_2)*(E1*Uinv) + a1*(E2*ac1*B1*u1)*(E1*dUinv_2) ;
dG12_3 = a1*(E2*ac1*B1*du1_3)*(E1*Uinv) + a1*(E2*ac1*B1*u1)*(E1*dUinv_3) ;
%dG12= dG12_1*dalpha1 + dG12_2*dalpha2 + dG12_3*dalpha3 ;

% D) Calcule de dG13_i
dG13_1 = a1*(E2*dac1_1*B1*u1 +E2*ac1*B1*du1_1)*(E1*Uinv) + a1*(E2*ac1*B1*u1)*(E1*dUinv_1) + a2*E2*dac1_1*B1 ;
dG13_2 = a1*(E2*ac1*B1*du1_2)*(E1*Uinv) + a1*(E2*ac1*B1*u1)*(E1*dUinv_2) ;
dG13_3 = a1*(E2*ac1*B1*du1_3)*(E1*Uinv) + a1*(E2*ac1*B1*u1)*(E1*dUinv_3) ;
%dG13= dG13_1*dalpha1 + dG13_2*dalpha2 + dG13_3*dalpha3 ;


% ----------------------------- Les deriveees partielles de Ca1 --------------------------------------

% 1) par rapport au d2alphai
dCa1_d2alpha1 = J1 + G13*dOC1_1 + G11*d_d2P_d2alpha1 ;
dCa1_d2alpha2 = G12*dOC2_2 + G11*d_d2P_d2alpha2 ;
dCa1_d2alpha3 = G12*dOC3_3 + G11*d_d2P_d2alpha3 ;
dCa1_d2alpha =[dCa1_d2alpha1 ,dCa1_d2alpha2 , dCa1_d2alpha3] ;

% 2) par rapport au dalphai
dCa1_dalpha1 = 2*G13*d2OC1_1*dalpha1 + G11*d_d2P_dalpha1 ;
dCa1_dalpha2 = 2*G12*d2OC2_2*dalpha2 + G11*d_d2P_dalpha2 ;
dCa1_dalpha3 = 2*G12*d2OC3_3*dalpha3 + G11*d_d2P_dalpha3 ;
dCa1_dalpha =[dCa1_dalpha1 ,dCa1_dalpha2 , dCa1_dalpha3] ;

% 3) par rapport au alphai 
dCa1_alpha1 = dG13_1*d2OC1 + G13*d_d2OC1_alpha1 + dG12_1*(d2OC2 + d2OC3) + dG11_1*d2P + G11*d_d2P_alpha1 ;
dCa1_alpha2 =  dG13_2*d2OC1 +  dG12_2*(d2OC2 + d2OC3) + G12*d_d2OC2_alpha2 + dG11_2*d2P + G11*d_d2P_alpha2 ;
dCa1_alpha3 =  dG13_3*d2OC1 +  dG12_3*(d2OC2 + d2OC3) + G12*d_d2OC3_alpha3 + dG11_3*d2P + G11*d_d2P_alpha3 ;
dCa1_alpha =[dCa1_alpha1 ,dCa1_alpha2 , dCa1_alpha3] ;

% test 
%dCa1 = dCa1_alpha*Dalpha +  dCa1_dalpha*Ddalpha + dCa1_d2alpha*Dd2alpha ;



%% ----------------------------- Linreairisation de Ca2 --------------------------------------

% A) la derivee de aci par rapport au ac2 :
dac2_2=[         0             l1*cos(alpha2)           0 
        -l1*cos(alpha2)            0             l1*sin(alpha2) 
                 0              -l1*sin(alpha2)          0                 ]   ;   
% B) Calcule de dG21_i
dG21_1 = a3*(E2*ac2*B2*du2_1)*(E2*Uinv) + a3*(E2*ac2*B2*u2)*(E2*dUinv_1) ;
dG21_2 = a3*(E2*dac2_2*B2*u2 +E2*ac2*B2*du2_2)*(E2*Uinv) + a3*(E2*ac2*B2*u2)*(E2*dUinv_2) + a1*E2*dac2_2*B2 ;
dG21_3 = a3*(E2*ac2*B2*du2_3)*(E2*Uinv) + a3*(E2*ac2*B2*u2)*(E2*dUinv_3) ;
%dG21= dG21_1*dalpha1 + dG21_2*dalpha2 + dG21_3*dalpha3 ;

G22=a1*(E2*ac2*B2*u2)*(E2/U)  ;
% C) Calcule de dG22_i
dG22_1 = a1*(E2*ac2*B2*du2_1)*(E2*Uinv) +  a1*(E2*ac2*B2*u2)*(E2*dUinv_1) ;
dG22_2 = a1*(E2*dac2_2*B2*u2 +E2*ac2*B2*du2_2)*(E2*Uinv) +a1*(E2*ac2*B2*u2)*(E2*dUinv_2) ;
dG22_3 = a1*(E2*ac2*B2*du2_3)*(E2*Uinv) + a1*(E2*ac2*B2*u2)*(E2*dUinv_3) ;
%dG22= dG22_1*dalpha1 + dG22_2*dalpha2 + dG22_3*dalpha3 ;

% D) Calcule de dG23_i
dG23_1 = a1*(E2*ac2*B2*du2_1)*(E2*Uinv) + a1*(E2*ac2*B2*u2)*(E2*dUinv_1) ;
dG23_2 = a1*(E2*dac2_2*B2*u2 +E2*ac2*B2*du2_2)*(E2*Uinv) + a1*(E2*ac2*B2*u2)*(E2*dUinv_2) + a2*E2*dac2_2*B2 ;
dG23_3 = a1*(E2*ac2*B2*du2_3)*(E2*Uinv) + a1*(E2*ac2*B2*u2)*(E2*dUinv_3) ;
%dG23= dG23_1*dalpha1 + dG23_2*dalpha2 + dG23_3*dalpha3 ;

% ----------------------------- Les deriveees partielles de Ca2 --------------------------------------

% 1) par rapport au d2alphai
dCa2_d2alpha2 = J1 + G23*dOC2_2 + G21*d_d2P_d2alpha2 ;
dCa2_d2alpha1 = G22*dOC1_1 + G21*d_d2P_d2alpha1 ;
dCa2_d2alpha3 = G22*dOC3_3 + G21*d_d2P_d2alpha3 ;
dCa2_d2alpha =[dCa2_d2alpha1 ,dCa2_d2alpha2 , dCa2_d2alpha3] ;

% 2) par rapport au dalphai
dCa2_dalpha1 = 2*G22*d2OC1_1*dalpha1 + G21*d_d2P_dalpha1 ;
dCa2_dalpha2 = 2*G23*d2OC2_2*dalpha2 + G21*d_d2P_dalpha2 ;
dCa2_dalpha3 = 2*G22*d2OC3_3*dalpha3 + G21*d_d2P_dalpha3 ;
dCa2_dalpha =[dCa2_dalpha1 ,dCa2_dalpha2 , dCa2_dalpha3] ;

% 3) par rapport au alphai 
dCa2_alpha1 =  dG23_1*d2OC2 +  dG22_1*(d2OC1 + d2OC3) + G22*d_d2OC1_alpha1 + dG21_1*d2P + G21*d_d2P_alpha1 ;
dCa2_alpha2 =  dG23_2*d2OC2 +  G23*d_d2OC2_alpha2 + dG22_2*(d2OC1 + d2OC3) + dG21_2*d2P + G21*d_d2P_alpha2 ;
dCa2_alpha3 =  dG23_3*d2OC2 +  dG22_3*(d2OC1 + d2OC3) + G22*d_d2OC3_alpha3 + dG21_3*d2P + G21*d_d2P_alpha3 ;
dCa2_alpha =[dCa2_alpha1 ,dCa2_alpha2 , dCa2_alpha3] ;

% test 
%dCa2 = dCa2_alpha*Dalpha +  dCa2_dalpha*Ddalpha + dCa2_d2alpha*Dd2alpha ;

%% ----------------------------- Linreairisation de Ca3 --------------------------------------

% A) la derivee de aci par rapport au ac3 :
dac3_3=[         0             l1*cos(alpha3)           0 
        -l1*cos(alpha3)            0             l1*sin(alpha3) 
                 0              -l1*sin(alpha3)          0                 ]   ;   


% B) Calcule de dG11_i
dG31_1 = a3*(E2*ac3*B3*du3_1)*(E3*Uinv) + a3*(E2*ac3*B3*u3)*(E3*dUinv_1) ;
dG31_2 = a3*(E2*ac3*B3*du3_2)*(E3*Uinv) + a3*(E2*ac3*B3*u3)*(E3*dUinv_2) ;
dG31_3 = a3*(E2*dac3_3*B3*u3 +E2*ac3*B3*du3_3)*(E3*Uinv) + a3*(E2*ac3*B3*u3)*(E3*dUinv_3) + a1*E2*dac3_3*B3 ;
%dG31= dG31_1*dalpha1 + dG31_2*dalpha2 + dG31_3*dalpha3 ;

% C) Calcule de dG12_i
dG32_1 = a1*(E2*ac3*B3*du3_1)*(E3*Uinv) + a1*(E2*ac3*B3*u3)*(E3*dUinv_1) ;
dG32_2 = a1*(E2*ac3*B3*du3_2)*(E3*Uinv) + a1*(E2*ac3*B3*u3)*(E3*dUinv_2) ;
dG32_3 = a1*(E2*dac3_3*B3*u3 +E2*ac3*B3*du3_3)*(E3*Uinv) + a1*(E2*ac3*B3*u3)*(E3*dUinv_3) ;
%dG32= dG32_1*dalpha1 + dG32_2*dalpha2 + dG32_3*dalpha3 ;

% D) Calcule de dG13_i
dG33_1 = a1*(E2*ac3*B3*du3_1)*(E3*Uinv) + a1*(E2*ac3*B3*u3)*(E3*dUinv_1) ;
dG33_2 = a1*(E2*ac3*B3*du3_2)*(E3*Uinv) + a1*(E2*ac3*B3*u3)*(E3*dUinv_2) ;
dG33_3 = a1*(E2*dac3_3*B3*u3 +E2*ac3*B3*du3_3)*(E3*Uinv) + a1*(E2*ac3*B3*u3)*(E3*dUinv_3) + a2*E2*dac3_3*B3 ;
%dG33= dG33_1*dalpha1 + dG33_2*dalpha2 + dG33_3*dalpha3 ;


% ----------------------------- Les deriveees partielles de Ca3 --------------------------------------

% 1) par rapport au d2alphai
dCa3_d2alpha1 = G32*dOC1_1 + G31*d_d2P_d2alpha1 ;
dCa3_d2alpha2 = G32*dOC2_2 + G31*d_d2P_d2alpha2 ;
dCa3_d2alpha3 = J1 + G33*dOC3_3 + G31*d_d2P_d2alpha3 ;
dCa3_d2alpha =[dCa3_d2alpha1 ,dCa3_d2alpha2 , dCa3_d2alpha3] ;

% 2) par rapport au dalphai
dCa3_dalpha1 = 2*G32*d2OC1_1*dalpha1 + G31*d_d2P_dalpha1 ;
dCa3_dalpha2 = 2*G32*d2OC2_2*dalpha2 + G31*d_d2P_dalpha2 ;
dCa3_dalpha3 = 2*G33*d2OC3_3*dalpha3 + G31*d_d2P_dalpha3 ;
dCa3_dalpha =[dCa3_dalpha1 ,dCa3_dalpha2 , dCa3_dalpha3] ;

% 3) par rapport au alphai 
dCa3_alpha1 =  dG33_1*d2OC3 +  dG32_1*(d2OC2 + d2OC1) + G32*d_d2OC1_alpha1 + dG31_1*d2P + G31*d_d2P_alpha1;
dCa3_alpha2 =  dG33_2*d2OC3 +  dG32_2*(d2OC2 + d2OC1) + G32*d_d2OC2_alpha2 + dG31_2*d2P + G31*d_d2P_alpha2 ;
dCa3_alpha3 = dG33_3*d2OC3 + G33*d_d2OC3_alpha3 + dG32_3*(d2OC2 + d2OC1) + dG31_3*d2P + G31*d_d2P_alpha3 ;
dCa3_alpha =[dCa3_alpha1 ,dCa3_alpha2 , dCa3_alpha3] ;

% test 
%dCa3 = dCa3_alpha*Dalpha +  dCa3_dalpha*Ddalpha + dCa3_d2alpha*Dd2alpha ;

%% Les derivees partielles de Ca ;

dCa_alpha = [dCa1_alpha;dCa2_alpha; dCa3_alpha] ;
dCa_dalpha = [dCa1_dalpha;dCa2_dalpha; dCa3_dalpha] ;
dCa_d2alpha = [dCa1_d2alpha;dCa2_d2alpha; dCa3_d2alpha] ;

%% Les derivees partielles de T par rapport au Theta ;
Theta = alpha*12 ; dTheta=dalpha*12 ; d2Theta = d2alpha*12; d3Theta=d3alpha*12;
dT_Theta = dCa_alpha/12^2 - dTg_Theta   ;
dT_dTheta = dCa_dalpha/12^2  ;
dT_d2Theta = dCa_d2alpha/12^2  ;
%  -----
T = Ta-Tg ;
 dT= dT_Theta*dTheta+dT_dTheta*d2Theta +dT_d2Theta*d3Theta ;

== matlab function Commande_2_BackStepping/RDelta_analityque/MDD/MDD/d2P par Calcule inverse /MCI ==
  data: P input; dP input; dP_alpha output; DH output
    function [dP_alpha,DH]= fcn(P,dP)

    l1 = 0.19992; 
    l2 = 0.334; 
    r = 0.126; 
    phi2 = 2*pi/3;
    phi3 = 4*pi/3;

    %% Expression de P dans Ri
    % l'expression P1 dP1 et d2P1 ne se changent pas
    A2=[cos(phi2) sin(phi2) 0
        -sin(phi2) cos(phi2) 0
        0            0      1 ]; 
    A3=[cos(phi3) sin(phi3) 0
        -sin(phi3) cos(phi3) 0
        0            0      1 ];
     P2=A2*P; dP2=A2*dP; 
     P3=A3*P ; dP3=A3*dP ; 
        
    x1=P(1); y1=P(2) ; z1=P(3) ; 
    x2=P2(1); y2=P2(2) ; z2=P2(3) ;
    x3=P3(1); y3=P3(2) ; z3=P3(3) ;
   
    %% Parametres du Triangle AiCiBi :
    % Triangle 1 :
    AB1=sqrt(z1^2+(x1-r)^2);
    e1=sqrt(l2^2-y1^2); 
    AB2=sqrt(z2^2+(x2-r)^2);
    e2=sqrt(l2^2-y2^2);
    AB3=sqrt(z3^2+(x3-r)^2);
    e3=sqrt(l2^2-y3^2);

    %% calcul de alpha1
    beta1=atan2(-z1,x1-r);
    delta1=acos((AB1^2 + l1^2 - e1^2)/(2*l1*AB1));
    alpha1=beta1-delta1; 


    %% calcul de alpha2
    beta2=atan2(-z2,x2-r);
    delta2=acos((AB2^2 + l1^2 - e2^2)/(2*l1*AB2));
    alpha2=beta2-delta2; 


    %% calcul de alpha3
    beta3=atan2(-z3,x3-r);
    delta3=acos((AB3^2 + l1^2 - e3^2)/(2*l1*AB3));
    alpha3=beta3-delta3; 

% Tranformation au Deg
alpha=[alpha1;alpha2;alpha3]; % first solution


%% =================== Calcule de dalpha_i ====================================

% ---------------------------- Calcul de dAlpha1 ----------------------
% Calcule de dDelta1 :
BH1 = AB1-l1*cos(delta1);
D1=l1*AB1*sin(delta1) ;
dDelta1X = -BH1*(x1-r)/AB1/D1 ; 
dDelta1Y = -y1/D1 ; 
dDelta1Z = -BH1*z1/AB1/D1 ; 
Gdelta1=  [ dDelta1X , dDelta1Y , dDelta1Z] ;
dDelta1 = Gdelta1*dP ;
% Calcule de dBeta1 :
dBeta1Z=-(x1-r)/AB1^2 ; dBeta1X=z1/AB1^2 ;
Gbeta1=[ dBeta1X ,  0 , dBeta1Z] ;
dBeta1 = Gbeta1*dP;
% Calcule de dAlpha1 :
Galpha1=Gbeta1-Gdelta1 ;
dAlpha1 = Galpha1*dP ;

% ---------------------------- Calcul de dAlpha2 ----------------------
% Calcule de dDelta2 :
BH2 = AB2-l1*cos(delta2);
D2=l1*AB2*sin(delta2) ;
dDelta2X = -BH2*(x2-r)/AB2/D2 ; 
dDelta2Y = -y2/D2 ; 
dDelta2Z = -BH2*z2/AB2/D2 ; 
Gdelta2=  [ dDelta2X , dDelta2Y , dDelta2Z] ;
dDelta2 = Gdelta2*dP2 ;
% Calcule de dBeta2 :
dBeta2Z=-(x2-r)/AB2^2 ; dBeta2X=z2/AB2^2 ;
Gbeta2=[ dBeta2X ,  0 , dBeta2Z] ;
dBeta2 = Gbeta2*dP2;
% Calcule de dAlpha2 :
Galpha2=Gbeta2-Gdelta2 ;
dAlpha2 = Galpha2*dP2 ;

% ---------------------------- Calcul de dAlpha3 ----------------------
% Calcule de dDelta2 :
BH3 = AB3-l1*cos(delta3);
D3=l1*AB3*sin(delta3) ;
dDelta3X = -BH3*(x3-r)/AB3/D3 ; 
dDelta3Y = -y3/D3 ; 
dDelta3Z = -BH3*z3/AB3/D3 ; 
Gdelta3=  [ dDelta3X , dDelta3Y , dDelta3Z] ;
dDelta3 = Gdelta3*dP3 ;
% Calcule de dBeta3:
dBeta3Z=-(x3-r)/AB3^2 ; dBeta2X=z3/AB3^2 ;
Gbeta3=[ dBeta2X ,  0 , dBeta3Z] ;
dBeta3 = Gbeta3*dP3;
% Calcule de dAlpha3 :
Galpha3=Gbeta3-Gdelta3 ;
dAlpha3 = Galpha3*dP3 ;

dalpha=[ dAlpha1 ; dAlpha2 ; dAlpha3 ];

%% ===================== Calcule de d2alpha_i =================================
 
% ---------------------------- Calcul de d2Alpha1 ----------------------
% Calcule de d2Gama1 :
CH1=l1*sin(delta1);
AH1=l1*cos(delta1) ;
d2Delta1XX = -BH1*(x1-r)^2/(AB1^3*D1)*( AH1*e1^2/(BH1*CH1^2) + (AB1/(x1-r))^2 - 2 ) ;
d2Delta1YY = - (1+y1^2*AH1*AB1/D1^2 )  /D1;
d2Delta1ZZ  = -BH1*z1^2/(AB1^3*D1)*( AH1*e1^2/(BH1*CH1^2) + (AB1/z1)^2 -2 ) ;
d2Delta1XY = y1*(x1-r)*(CH1^2-AH1*BH1)/D1^3 ;
d2Delta1XZ = -BH1*(x1-r)*z1/(AB1^3*D1)*( AH1*e1^2/(BH1*CH1^2) - 2 ) ;
d2Delta1YZ = y1*z1*(CH1^2-AH1*BH1)/D1^3 ; 
Hdelta1=[ d2Delta1XX,d2Delta1XY,d2Delta1XZ ; d2Delta1XY, d2Delta1YY,d2Delta1YZ ;d2Delta1XZ , d2Delta1YZ,d2Delta1ZZ] ;

%Calcule de dBeta 1:
d2Beta1XX=-2*(x1-r)*z1/AB1^4 ; d2Beta1ZZ=-d2Beta1XX ; d2Beta1XZ = ((x1-r)^2-z1^2)/AB1^4 ;
Hbeta1= [d2Beta1XX , 0, d2Beta1XZ ; 0, 0, 0 ; d2Beta1XZ , 0 , d2Beta1ZZ ] ;

%Calcule de dAlpha1 :
Halpha1= Hbeta1 - Hdelta1; 


% ---------------------------- Calcul de d2Alpha2 ----------------------
% Calcule de d2Gama1 :
CH2=l1*sin(delta2);
AH2=l1*cos(delta2) ;
d2Delta2XX = -BH2*(x2-r)^2/(AB2^3*D2)*( AH2*e2^2/(BH2*CH2^2) + (AB2/(x2-r))^2 - 2 ) ;
d2Delta2YY = - (1+y2^2*AH2*AB2/D2^2 )  /D2;
d2Delta2ZZ  = -BH2*z2^2/(AB2^3*D2)*( AH2*e2^2/(BH2*CH2^2) + (AB2/z2)^2 -2 ) ;
d2Delta2XY = y2*(x2-r)*(CH2^2-AH2*BH2)/D2^3 ;
d2Delta2XZ = -BH2*(x2-r)*z2/(AB2^3*D2)*( AH2*e2^2/(BH2*CH2^2) - 2 ) ;
d2Delta2YZ = y2*z2*(CH2^2-AH2*BH2)/D2^3 ; 
Hdelta2=[ d2Delta2XX,d2Delta2XY,d2Delta2XZ ; d2Delta2XY, d2Delta2YY,d2Delta2YZ ;d2Delta2XZ , d2Delta2YZ,d2Delta2ZZ] ;

%Calcule de dBeta2:
d2Beta2XX=-2*(x2-r)*z2/AB2^4 ; d2Beta2ZZ=-d2Beta2XX ; d2Beta2XZ = ((x2-r)^2-z2^2)/AB2^4 ;
Hbeta2= [d2Beta2XX , 0, d2Beta2XZ ; 0, 0, 0 ; d2Beta2XZ , 0 , d2Beta2ZZ ] ;

%Calcule de dAlpha2 :
Halpha2= Hbeta2 - Hdelta2; 


% ---------------------------- Calcul de d2Alpha3 ----------------------
% Calcule de d2Gama3 :
CH3=l1*sin(delta3);
AH3=l1*cos(delta3) ;
d2Delta3XX = -BH3*(x3-r)^2/(AB3^3*D3)*( AH3*e3^2/(BH3*CH3^2) + (AB3/(x3-r))^2 - 2 ) ;
d2Delta3YY = - (1+y3^2*AH3*AB3/D3^2 )  /D3;
d2Delta3ZZ  = -BH3*z3^2/(AB3^3*D3)*( AH3*e3^2/(BH3*CH3^2) + (AB3/z3)^2 -2 ) ;
d2Delta3XY = y3*(x3-r)*(CH3^2-AH3*BH3)/D3^3 ;
d2Delta3XZ = -BH3*(x3-r)*z3/(AB3^3*D3)*( AH3*e3^2/(BH3*CH3^2) - 2 ) ;
d2Delta3YZ = y3*z3*(CH3^2-AH3*BH3)/D3^3 ; 
Hdelta3=[ d2Delta3XX,d2Delta3XY,d2Delta3XZ ; d2Delta3XY, d2Delta3YY,d2Delta3YZ ;d2Delta3XZ , d2Delta3YZ,d2Delta3ZZ] ;

%Calcule de dBeta3:
d2Beta3XX=-2*(x3-r)*z3/AB3^4 ; d2Beta3ZZ=-d2Beta3XX ; d2Beta3XZ = ((x3-r)^2-z3^2)/AB3^4 ;
Hbeta3= [d2Beta3XX , 0, d2Beta3XZ ; 0, 0, 0 ; d2Beta3XZ , 0 , d2Beta3ZZ ] ;

%Calcule de dAlpha3 :
Halpha3= Hbeta3 - Hdelta3; 


 % d2alpha=[d2Alpha1 ; d2Alpha2 ; d2Alpha3]; ou bien :

H = [dP'*Halpha1*dP ;dP2'*Halpha2*dP2 ;dP3'*Halpha3*dP3 ] ;
D = [Galpha1;Galpha2*A2;Galpha3*A3] ;
dP_alpha =eye(3)/D ;
DH = D\H ;
%% Clacule inverse de d2P :

% d2P =D\d2alpha-D\H ;

== matlab function Commande_2_BackStepping/RDelta_analityque/MDD/MDD/d2P par calcule inverse ==
  data: alpha input; dalpha input; dP_alpha input; DH input; d2alpha output; Cg input; T input; P input; M output; N output
function [d2alpha, M,N]= fcn(alpha,dalpha, dP_alpha,DH,Cg,T,P)

alpha1=alpha(1) ;alpha2=alpha(2) ; alpha3=alpha(3) ;
dalpha1=dalpha(1) ;dalpha2=dalpha(2) ; dalpha3=dalpha(3) ;

%% les constantes
    l1 = 0.19992; 
    l2 = 0.334; 
    r = 0.126; 
    phi2 = 2*pi/3;
    phi3 = 4*pi/3;
A2=[cos(phi2) sin(phi2) 0
    -sin(phi2) cos(phi2) 0
    0            0      1 ]; 
A3=[cos(phi3) sin(phi3) 0
    -sin(phi3) cos(phi3) 0
    0            0      1 ];
% Constantes mecaniques
    J1=0.0071126;
    M2=2*0.01438  ;
    J2 = 2*0.00027499613;
    M3 = 0.04157 ;
    M4=2*J2/l2^2 ;
    
% Fin

% les vecteurs OAi et OCi :
OC1=[r+l1*cos(alpha1) ; 0 ; -l1*sin(alpha1) ]; 
OC2=[(r+l1*cos(alpha2))*cos(phi2) ; (r+l1*cos(alpha2))*sin(phi2) ; -l1*sin(alpha2) ]; 
OC3=[(r+l1*cos(alpha3))*cos(phi3) ; (r+l1*cos(alpha3))*sin(phi3) ; -l1*sin(alpha3) ]; 
%fin

% Les vecteurs unitaires portes par les bras paralleles : la nouvelle base
u1=(P-OC1)/l2 ; u2=(P-OC2)/l2 ; u3=(P-OC3)/l2 ;
%la matrice du transformation = La nouvelle base:
U = [u1 u2 u3] ;
%Uinv=inv(U);

%%  accelerations des points Ci :
% dOCi : la derivee partielle de OCi par rapport au alphai
% d2OCi : la deuxieme derivee partielle de OCi par rapport au alphai

dOC1_1=[-l1*sin(alpha1) ; 0 ; -l1*cos(alpha1)] ; 
dOC2_2=[-l1*sin(alpha2)*cos(phi2) ; -l1*sin(alpha2)*sin(phi2) ; -l1*cos(alpha2)] ;
dOC3_3=[-l1*sin(alpha3)*cos(phi3) ; -l1*sin(alpha3)*sin(phi3) ; -l1*cos(alpha3)] ;

d2OC1_1=[-l1*cos(alpha1) ; 0 ; l1*sin(alpha1)] ;
d2OC2_2=[-l1*cos(alpha2)*cos(phi2) ; -l1*cos(alpha2)*sin(phi2) ; l1*sin(alpha2)] ;
d2OC3_3=[-l1*cos(alpha3)*cos(phi3) ; -l1*cos(alpha3)*sin(phi3) ; l1*sin(alpha3)] ;

%Fin

%% ================ Le couple Cai en point de fonctionnement Couple1==================
% Parametres:
a1 = M2/4-M4/2 ; a2= M2/4 + M4/2; a3=M3 +3*a2 ; 
% la matrice de cross(AiCi,...)=aci  "ACi est exprimee dans le repere Ri"
ac1=[ 0 , l1*sin(alpha1) , 0 ; -l1*sin(alpha1) ,0 , -l1*cos(alpha1) ; 0 , l1*cos(alpha1),0]   ;
ac2=[ 0 , l1*sin(alpha2) , 0 ; -l1*sin(alpha2) ,0 , -l1*cos(alpha2) ; 0 , l1*cos(alpha2),0]   ;
ac3=[ 0 , l1*sin(alpha3) , 0 ; -l1*sin(alpha3) ,0 , -l1*cos(alpha3) ; 0 , l1*cos(alpha3),0]   ;
% Les matrices de projection
E1 = [1 0 0]; E2 = [0 1 0]; E3 = [0 0 1];
B1= [1 0 0; 0 0 0 ; 0 0 1] ; B2=B1*A2; B3=B1*A3 ;
%% 1)  Le couple Ca1 : 
G11=a3*(E2*ac1*B1*u1)*(E1/U) + a1*E2*ac1*B1 ;
G12=a1*(E2*ac1*B1*u1)*(E1/U)  ;
G13=a1*(E2*ac1*B1*u1)*(E1/U) + a2*E2*ac1*B1 ;
%Ca1=(J1+G13*dOC1_1)*d2alpha1+ G11*d2P +(G12*dOC2_2)*d2alpha2 + (G12*dOC3_3)*d2alpha3 +G13*d2OC1_1*dalpha1^2+ (G12*d2OC2_2)*dalpha2^2 + (G12*d2OC3_3)*dalpha3^2;
% Ca1 = J1*d2alpha1 + G11*d2P + G12* (d2OC2 +d2OC3) + G13*d2OC1 ;

%% 2)  Le couple Ca2 : 
G21=a3*(E2*ac2*B2*u2)*(E2/U) + a1*E2*ac2*B2 ;
G22=a1*(E2*ac2*B2*u2)*(E2/U)  ;
G23=a1*(E2*ac2*B2*u2)*(E2/U) + a2*E2*ac2*B2 ;
%Ca2=(J1+G23*dOC2_2)*d2alpha2+ G21*d2P +(G22*dOC1_1)*d2alpha1 + (G22*dOC3_3)*d2alpha3 +G23*d2OC2_2*dalpha2^2+ (G22*d2OC1_1)*dalpha1^2 + (G22*d2OC3_3)*dalpha3^2;
%Ca2 = J1*d2alpha2 + G21*d2P + G22* (d2OC1 +d2OC3) + G23*d2OC2 ;

%% 3)  Le couple Ca3 : 
G31=a3*(E2*ac3*B3*u3)*(E3/U) + a1*E2*ac3*B3 ;
G32=a1*(E2*ac3*B3*u3)*(E3/U)  ;
G33=a1*(E2*ac3*B3*u3)*(E3/U) + a2*E2*ac3*B3 ;
%Ca3=(J1+G33*dOC3_3)*d2alpha3+ G31*d2P +(G32*dOC2_2)*d2alpha2 + (G32*dOC1_1)*d2alpha1 + G33*d2OC3_3*dalpha3^2+ (G32*d2OC2_2)*dalpha2^2 + (G32*d2OC1_1)*dalpha1^2;
% Ca3 = J1*d2alpha3 + G31*d2P + G32* (d2OC2 +d2OC1) + G33*d2OC3 ;
% Fin

 %% ============= Calcule inverse de MDD (d2alpha en fonction de Ca ===========

e11= J1+G13*dOC1_1 ; 
e12 = (G12*dOC2_2) ;
e13 = (G12*dOC3_3) ;
b11 = G13*d2OC1_1 ;
b12 = (G12*d2OC2_2) ;
b13 =(G12*d2OC3_3) ;
% Ca1=e11*d2alpha1+e12*d2alpha2 + e13*d2alpha3 +b11*dalpha1^2+ b12*dalpha2^2 + b13*dalpha3^2 + G11*d2P ;

e21 = (G22*dOC1_1) ;
e22 = (J1+G23*dOC2_2) ;
e23 = (G22*dOC3_3) ;
b21 = (G22*d2OC1_1) ;
b22 = G23*d2OC2_2 ;
b23 = (G22*d2OC3_3) ;
% Ca2 = e22*d2alpha2 + e21*d2alpha1 + e23*d2alpha3 +b22*dalpha2^2 + b21*dalpha1^2 + b23*dalpha3^2 + G21*d2P ;

e31 = (G32*dOC1_1) ;
e32 =(G32*dOC2_2) ;
e33 =(J1+G33*dOC3_3);
b31 = (G32*d2OC1_1) ;
b32 =(G32*d2OC2_2) ;
b33 = G33*d2OC3_3 ;
% Ca3=e33*d2alpha3 +e32*d2alpha2 + e31*d2alpha1 + b33*dalpha3^2+ b32*dalpha2^2 + b31*dalpha1^2 + G31*d2P;

e=[e11 , e12 , e13 ; e21 , e22 , e23 ; e31 , e32 , e33] ;
b=[b11 , b12, b13 ; b21 , b22 , b23 ; b31, b32, b33] ;
G = [G11 ; G21 ; G31]  ;
dalphaCarre=[dalpha1^2 ; dalpha2^2; dalpha3^2] ;
% Ca = e*d2alpha + b*dalphaCarre + G*d2P ;
N = 12^2*eye(3,3)/(e+G*dP_alpha);
M = (e+G*dP_alpha)\(Cg - b*dalphaCarre + G*DH)*12 ;

%% Calcule de d2alpha :
%Ca=12*T +Cg ;
%d2alpha =(e+G*dP_alpha)\12*T +(e+G*dP_alpha)\(Cg  - b*dalphaCarre + G*DH) ; 
d2Theta = M + N*T ;
d2alpha = d2Theta /12 ;

== matlab function Commande_2_BackStepping/RDelta_analityque/MDD/MG le  nouveau ==
  data: alpha input; P output
function P =MGD(alpha)


alpha1=alpha(1) ;alpha2=alpha(2) ; alpha3=alpha(3) ;

%les constantes
l1 = 0.19992; 
l2 = 0.334; 
r = 0.126; 
phi2 = 2*pi/3;
phi3 = 4*pi/3;

%% Les points :
C1=[r+l1*cos(alpha1) ; 0 ; -l1*sin(alpha1) ]; 
C2=[(r+l1*cos(alpha2))*cos(phi2) ; (r+l1*cos(alpha2))*sin(phi2) ; -l1*sin(alpha2) ]; 
C3=[(r+l1*cos(alpha3))*cos(phi3) ; (r+l1*cos(alpha3))*sin(phi3) ; -l1*sin(alpha3) ]; 

%% Les vecteurs du triangle C1C2C3 et ses distances
C1C2= C2-C1 ; C2C3 =C3-C2 ; C3C1= C1-C3 ;
a=sqrt(C1C2'*C1C2) ; b=sqrt(C2C3'*C2C3)  ; c=sqrt(C3C1'*C3C1)  ;
 p= a+b+c ; % Le perimetre de C1C2C3
 R = a*b*c/sqrt(p*(p-2*a)*(p-2*b)*(p-2*c)) ;

 %% Calcule du point L 
 % Les vecteurs u et n:
 v1=C1C2/a ;
 n=cross(C3C1,C1C2)*2*R/(a*b*c) ;
 TL = sqrt(R^2-a^2/4) ;
 OL=(C1+C2)/2+TL*sign(-a*a+c*c+b*b)*cross(n,v1);
 %% Calcule du point E :
P=OL-sqrt(l2^2-R^2)*n ;

== matlab function Commande_2_BackStepping/Trajectoir ==
  data: t input; ne input; P output; dP output; d2P output; d3P output
function [P,dP,d2P,d3P]= fcn(t,ne)

%% Menu
% 1 ==> Ligne horizontal
% 2==>  Ligne suivant l'axe oz
% 3==> Cercle
% 4==> Ligne x=y
 z0=-0.08789 ; zpi=-0.3;
B= (z0+zpi)/2 ; A= (z0-zpi)/2 ; 
f = 3; f2 = 5 ;
R=0.2;
%% vers le Plan Z=-0.3
if (t<pi/f && (ne == 1 || ne == 3 ||  ne == 0 || ne == 4 || ne == 5 ||  ne == 6))
n= 2 ; 
elseif( (ne == 4 || ne == 5 ||  ne == 6)  &&  (t<3*pi/2/f) ) % vers le point (0 , R , -0.3)
n=1 ;
else
n =ne ;
end

%% le trajecoir
switch n
    
    case 0
        
        % La position
        x = R*sin(f*t)  ; y=0 ;
        z=  zpi ;
        P = [ x ; y ; z ];
        % La vitess
        dx = f*R*cos(f*t)  ; dy=0 ;
        dz= 0 ;
        dP = [ dx ; dy ; dz ];
        % L'acceleration :
        d2x = -f^2*R*sin(f*t) ; d2y=0 ;
        d2z =  0;
        d2P = [ d2x ; d2y ; d2z ];
        % L'a _coup :
        d3x = -f^3*R*cos(f*t) ; d3y=0 ;
        d3z =  0;
        d3P = [ d3x ; d3y ; d3z ];
    case 1   
        % La position
        y = R*sin(f*t)  ; x=0 ;
        z= zpi  ;
        P = [ x ; y ; z ];
        % La vitess
        dy = f*R*cos(f*t)  ; dx=0 ;
        dz= 0 ;
        dP = [ dx ; dy ; dz ];
        % L'acceleration :
        d2y = -f^2*R*sin(f*t) ; d2x=0 ;
        d2z =  0;
        d2P = [ d2x ; d2y ; d2z ];
        % L'a _coup :
        d3y = -f^3*R*cos(f*t) ; d3x=0 ;
        d3z =  0;
        d3P = [ d3x ; d3y ; d3z ];
    case 2
        % La position 
        x = 0 ; y=0 ;
        z= A*cos(f*t) + B ; 
        P = [ x ; y ; z ];
        % La vitess
        dx = 0 ; dy=0 ;
        dz= -f*A*sin(f*t) ;
        dP = [ dx ; dy ; dz ];
        % L'acceleration :
        d2x = 0 ; d2y=0 ;
        d2z = -f^2*A*cos(f*t) ;
        d2P = [ d2x ; d2y ; d2z ];
        % L a_coup (jerk) :
        d3x = 0 ; d3y=0 ;
        d3z = f^3*A*sin(f*t) ;
        d3P = [ d3x ; d3y ; d3z ];
        
        %%
    case 3
        R=0.12;
        y = R*sin(f*t)  ; x=2*y;
        z= zpi  ;
        P = [ x ; y ; z ];
        % La vitess
        dy = f*R*cos(f*t)  ; dx=2*dy ;
        dz= 0 ;
        dP = [ dx ; dy ; dz ];
        % L'acceleration :
        d2y = -f^2*R*sin(f*t) ; d2x=2*d2y ;
        d2z =  0;
        d2P = [ d2x ; d2y ; d2z ];
        % L'a _coup :
        d3y = -f^3*R*cos(f*t) ; d3x=2*d3y ;
        d3z =  0;
        d3P = [ d3x ; d3y ; d3z ];
    case 4 % Cerecl XY
        x=R*cos(f*t) ; y=R*sin(f*t) ; z=zpi  ;
        dx=-f*R*sin(f*t) ; dy=f*R*cos(f*t)  ;  dz=0;
        d2x=-f^2*R*cos(f*t) ; d2y=-f^2*R*sin(f*t)  ;  d2z=0;
        P=[x ; y ; z];
        dP=[dx ; dy ; dz];
        d2P=[d2x ; d2y ; d2z];
        % L'a _coup :
        d3x=f^3*R*sin(f*t) ; d3y=-f^3*R*cos(f*t)  ;  d3z=0;
        d3P=[d3x ; d3y ; d3z];
        
    case 5 % ZY   
        x=0 ; y=R*sin(f*t) ; z=0.5*R*cos(f*t) + zpi  ;
        dx=0 ; dy=f*R*cos(f*t)  ;  dz=-f*0.5*R*sin(f*t);
        d2x=0 ; d2y=-f^2*R*sin(f*t)  ;  d2z=-f^2*0.5*R*cos(f*t);
        P=[x ; y ; z];
        dP=[dx ; dy ; dz];
        d2P=[d2x ; d2y ; d2z];
        d3x=0 ; d3y=-f^3*R*cos(f*t)  ;  d3z=f^3*0.5*R*sin(f*t);
        d3P=[d3x ; d3y ; d3z];
%     case 6 %Cercle ZX
%         y=0 ; x=R*sin(f*t) ; z=R*cos(f*t) +zpi;
%         dy=0 ; dx=f*R*cos(f*t)  ;  dz=-f*R*sin(f*t);
%         d2y=0 ; d2x=-f^2*R*sin(f*t)  ;  d2z=-f^2*R*cos(f*t);
%         d3y=0 ; d3x=-f^3*R*cos(f*t)  ;  d3z=f^3*R*sin(f*t);
%         P=[x ; y ; z];
%         dP=[dx ; dy ; dz];
%         d2P=[d2x ; d2y ; d2z];
%         d3P = [ d3x ; d3y ; d3z ];
%     case 7  % Les derivees sont a corriger
%         R=0.00*sin(f2*t) ; A=0.1270 ;
%         x=R*cos(f*t) ; y=R*sin(f*t) ;
%         z= A*sin(f2*t) -0.2 ;
%         dx=-f*R*sin(f*t) ; dy=f*R*cos(f*t)  ;  
%         dz= f2*A*cos(f2*t) ;
%         d2x=-f^2*R*cos(f*t) ; d2y=-f^2*R*sin(f*t)  ;
%         d2z = -f2^2*A*sin(f2*t) ;
%         P=[x ; y ; z];
%         dP=[dx ; dy ; dz];
%         d2P=[d2x ; d2y ; d2z];
%         % L'a _coup :
%         d3x=f^3*R*sin(f*t) ; d3y=-f^3*R*cos(f*t)  ;
%         d3z = -f2^3*A*cos(f2*t) ;
%         d3P=[d3x ; d3y ; d3z];
    case 8
        x=0 ; y=0 ; z=z0 ;
        P=[x ; y ; z];
        dP=[0 ; 0 ; 0];
        d2P=[0 ; 0 ; 0];
        d3P=[0 ; 0 ; 0];
        
    otherwise
        P=[0 ; 0 ; 0];
        dP=[0 ; 0 ; 0];
        d2P=[0 ; 0 ; 0];
        d3P = [ 0 ; 0 ; 0 ];
end

== matlab function Commande_2_BackStepping/RDelta_analityque/Moteurs/equations electriques ==
  data: I input; U input; dI output; dTheta input
function dI = fcn(I,U,dTheta)

% Les Constantes des moteurs ;

b1 = -1.1250e+03 ;
b2 = -99.4718 ;
b3 =833.3333 ;

dI = b2*dTheta + b1*I + b3*U ;
